simulink model "PID"  (R2023b)
settings: Solver=VariableStepAuto  StartTime=0.0  StopTime=10.0  MaxStep=0.01  RelTol=1e-3
settings Model: Creator=jerry  LastModifiedBy=jerry

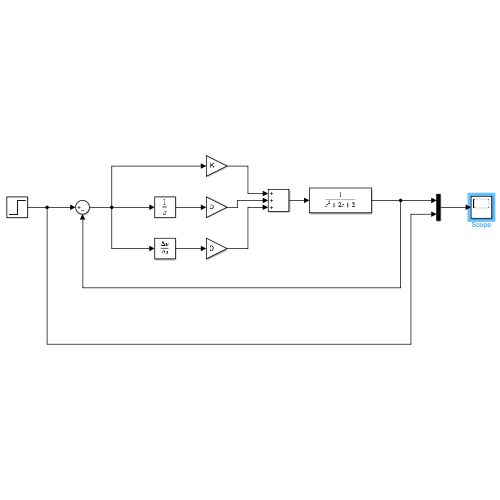
[thumbnail: Simulink's stored preview of the top-level diagram]
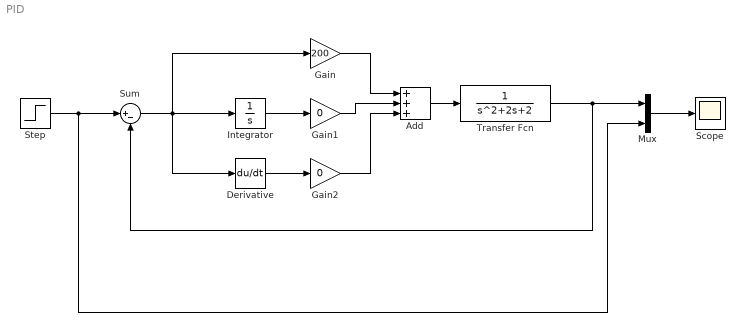
== system PID ==
  Add : Sum  Inputs=+++
  Derivative : Derivative
  Gain : Gain  Gain=200
  Gain1 : Gain  Gain=0
  Gain2 : Gain  Gain=0
  Integrator : Integrator
  Mux : Mux  Inputs=2
  Scope : Scope
  Step : Step  SampleTime=0
  Sum : Sum  Inputs=|+-
  Transfer Fcn : TransferFcn  Denominator=[1 2 2]
  wires:
  Gain2/1 -> Add/3
  Gain1/1 -> Add/2
  Gain/1 -> Add/1
  Integrator/1 -> Gain1/1
  Derivative/1 -> Gain2/1
  Sum/1 -> Derivative/1, Integrator/1, Gain/1
  Add/1 -> Transfer Fcn/1
  Transfer Fcn/1 -> Mux/1, Sum/2
  Mux/1 -> Scope/1
  Step/1 -> Mux/2, Sum/1
